simulink library "DeePC_lib"  (R2024b)
settings: Solver=VariableStepAuto  StartTime=0.0  StopTime=10.0  RelTol=1e-3
values from neighbouring files (symbols this model uses):
  Uf = U_hankel(T_ini+1:end, :)    [save_hankel_data_gemini.m]
  Up = U_hankel(1:T_ini, :)    [save_hankel_data_gemini.m]
  Yf = Y_hankel(T_ini+1:end, :)    [save_hankel_data_gemini.m]
  Yp = Y_hankel(1:T_ini, :)    [save_hankel_data_gemini.m]
settings Model: Creator=scherg  LastModifiedBy=scherg

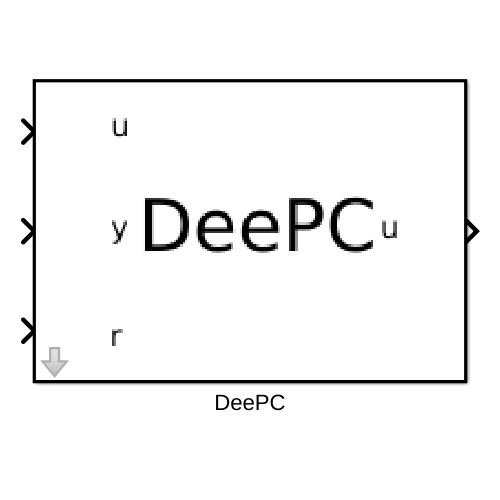
[thumbnail: Simulink's stored preview of the top-level diagram]
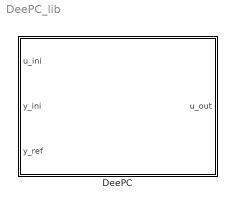
== system DeePC_lib ==
  DeePC : MATLAB Function  TreatAsAtomicUnit=on  mask{Up=Up, Yp=Yp, Uf=Uf, Yf=Yf, q=400, r=1, lambda=1e-4, u_limit=4.0}
      mask prompts: q "Higher Bandwidth Increase Q"; r "Better Smoothness Increase R"; lambda "larger lambda makes the controller more robust to disturbances and noise"; u_limit "Control signal limit (+-)"

== matlab function DeePC_lib/DeePC ==
  data: u_ini input size=[T_ini 1]; u_out output size=[1 1]; y_ini input size=[T_ini 1]; y_ref input size=[1 1]; Up parameter; Yp parameter; Uf parameter; Yf parameter; q parameter; r parameter; lambda parameter; u_limit parameter
function u_out = deepc_controller(u_ini, y_ini, y_ref, Up, Yp, Uf, Yf, q, r, lambda, u_limit)

    % u_ini: [Tini*m x 1] 
    % y_ini: [Tini*p x 1]
    % y_ref: [N*p x 1]
    % Up, Uf, Yp, Yf: Pre-partitioned Hankel matrices from offline data

    % --- Persistent Variables for Speed ---
    persistent G_mat x0_warm first_run m p N Tini u_prev u_f_sol Q R du_max du_min A_cons I_vec S
    
    % --- Initialization (t = 0) ---
    if isempty(first_run)
        [row_Up, ~] = size(Up);
        [row_Uf, ~] = size(Uf);
        [row_Yp, ~] = size(Yp);
        [row_Yf, ~] = size(Yf);
        
        m = 1; % Adjust to your number of inputs
        p = 1; % Adjust to your number of outputs
        Tini = row_Up / m;
        N = row_Uf / m;

        % Compute the "Image" of the data (the G matrix)
        % This projects the relationship into the input/output space
        % g_fixed = [Up; Yp; Uf] pinv * [u_ini; y_ini; u_f]
        % We pre-calculate the fundamental mapping:
        % --- 1. Disturbance Rejection Knob (Lambda) ---
        % lambda = 1e-4; % Increase this to 1e-2 if system is too "twitchy"
        H_offline = [Up; Yp; Uf];
        % Regularized pseudo-inverse
        H_pseudo = (H_offline' * H_offline + lambda * eye(size(H_offline,2))) \ H_offline';
        % H_pseudo = pinv([Up; Yp; Uf]); 
        G_mat = Yf * H_pseudo; 

        u_f_sol = zeros(N*m+1, 1); % plus slack

        % --- The Incremental Logic ---
        % u_f(k) = u(t-1) + sum_{i=1}^{k} delta_u(i)
        % We create a Summation Matrix 'S' to relate delta_u to absolute u_f
        % u_f = S * delta_u + I_vec * u_prev
        S = tril(ones(N*m)); 
        I_vec = ones(N*m, 1);
        A_cons = [S, -ones(N*m, 1); -S, -ones(N*m, 1)]; % Inequality matrix for absolute saturation with Slack Buffer

        % --- Weights (Tune these!) ---
        Q = eye(size(Yf, 1)) * q;  % Output tracking weight
        R = eye(size(Uf, 1)) * r;    % Control effort weight

        % --- Constraints ---
        % Example: du_min <= u_f <= du_max % Lower bound for slack: must be >= 0
        du_max = [3 * ones(N*m, 1); inf]; 
        du_min = [-3 * ones(N*m, 1); 0];
        
        % Initialize warm start vector for u_f (size N*m)
        x0_warm = zeros(N*m+1, 1);
        u_prev = 0;              % To track the absolute u applied
        first_run = 1;
        u_out = 0;
        return;
    end

    % Slack Weight (S_w): Must be MUCH larger than Q to keep constraints "hard"
    % until they absolutely must be broken.
    S_w = 1e6;

    % --- Construct Reduced QP ---
    % Standard DeePC: min ||Yf*g - y_ref||^2_Q + ||Uf*g||^2_R
    % Reduced: We express Yf*g as a function of u_f and initial conditions
    
    % Split the pre-calculated projection for the current [u_ini; y_ini]
    % Yf*g = G1*u_ini + G2*y_ini + G3*u_f
    G_const = G_mat(:, 1:size(Up,1)+size(Yp,1));
    G_v = G_mat(:, size(Up,1)+size(Yp,1)+1:end);
    % Fixed part of the prediction based on past data
    % y_fixed = G_const * [u_ini; y_ini];
    y_fixed = G_const * [u_ini; y_ini] + G_v * I_vec * u_prev;

    y_ref_vec = y_ref*ones(N,1);

    % Quadratic Programming form: 0.5*u_f'*H_qp*u_f + f_qp'*u_f
    M = G_v * S;
    % Augmented Hessian: H_total = [H_qp, 0; 0, S_w]
    H_qp_core = 2 * (M' * Q * M + R);
    H_qp = blkdiag(H_qp_core, S_w);
    % Augmented f: f_total = [f_qp; 0]
    f_qp_core = 2 * M' * Q * (y_fixed - y_ref_vec);
    f_qp = [f_qp_core; 0];
    
    % Force symmetry to satisfy quadprog
    H_qp = (H_qp + H_qp') / 2;

    % --- 2. Absolute Saturation Limits ---
    % u_limit = 4.0; % Example: throttle/steering limit
    % b_cons changes every step because it depends on u_prev
    b_cons = [u_limit * I_vec - I_vec * u_prev; 
              u_limit * I_vec + I_vec * u_prev];
    
    
    % --- Solver Options ---
    % 'active-set' is required for Simulink Code Generation
    opts = optimoptions('quadprog', 'Display', 'off', 'Algorithm', 'active-set');
    
    % Call Solver with Warm Start (x0_warm)
    coder.extrinsic('quadprog');
    
    exitflag = 0;
    
    [u_f_sol, ~, exitflag] = quadprog(H_qp, f_qp, A_cons, b_cons, [], [], du_min, du_max, x0_warm, opts);

    % --- Output and Warm Start Update ---
    if exitflag > 0
        % Apply the first control action
        delta_u_now = u_f_sol(1); %:m);
        u_out = u_prev + delta_u_now;
        
        % Update for next step
        u_prev = u_out;
        % Update Warm Start for next iteration (Shift-and-append)
        % We shift the solution one step and pad with the last value
        x0_warm = [u_f_sol(m+1:end-1); 0; u_f_sol(end)]; % Shift delta_u, keep slack %(m+1:end); u_f_sol(end-m+1:end)];
    else
        % If optimization fails, fallback to previous or zero
        u_out = u_prev;
    end
end

%     % u_ini: [T_ini x 1] vector of recent inputs
%     % y_ini: [T_ini x 1] vector of recent outputs
%     % y_ref: [N x 1] vector of desired future outputs
%     u_out = 0; % Pre-allocate so Simulink knows the type
%     persistent last_u H_mat f_vec Aeq n_vars x0
%     if isempty(last_u)
%         last_u = 0; 
%     end
% 
%     % Decision variable for quadprog: [g; sigma]
%     % We use the g-vector to span the signal space and sigma to handle noise
%     num_columns = size(Up, 2);
%     num_sigma = size(Yp, 1);
% 
%     % --- Cost Function Formulation ---
%     % We want to minimize: ||Yf*g - y_ref||^2_Q + ||Uf*g||^2_R + L_g*||g||^2 + L_s*||sigma||^2
%     % 0.5 * z' * H_mat * z + f_vec' * z
% 
%     if isempty(H_mat)
%         H_mat = blkdiag(2*(Yf'*Q*Yf + Uf'*R*Uf + lambda_g*eye(num_columns)), 2*lambda_sigma*eye(num_sigma));
%         H_mat = (H_mat + H_mat') / 2; % Ensure perfect symmetry for the solver
%         f_vec = [(-2*y_ref'*Q*Yf)'; zeros(num_sigma, 1)];
% 
%         % --- Equality Constraints ---
%         % [Up; Yp]*g + [0; sigma] = [u_ini; y_ini]
%         Aeq = [Up, zeros(size(Up, 1), num_sigma); 
%                Yp, eye(num_sigma)];
% 
%         n_vars = size(H_mat, 1);
%         x0 = zeros(n_vars, 1);
%     end
%     beq = [u_ini; y_ini];
% 
%     % --- Solving (Using interior-point for speed) ---
%     opts = optimoptions('quadprog', 'Display', 'off', 'Algorithm', 'active-set');
%     % Define the number of decision variables (usually g = size(U_p, 2))
% 
%     z_opt = quadprog(H_mat, f_vec, [], [], Aeq, beq, [], [], x0, opts);
% 
%     if isempty(z_opt)
%         u_out = last_u; % Fallback if optimization fails
%     else
%         g_opt = z_opt(1:num_columns);
%         u_future = Uf * g_opt;
%         u_out = u_future(1); % Apply first step (Receding Horizon)
%         last_u = u_out;
%     end
% end
